simulink model "Sim4"  (R2014a)
settings: Solver=ode45  StartTime=0.0  StopTime=10.0  RelTol=1e-3
settings Model: Creator=OCAC  LastModifiedBy=OCAC

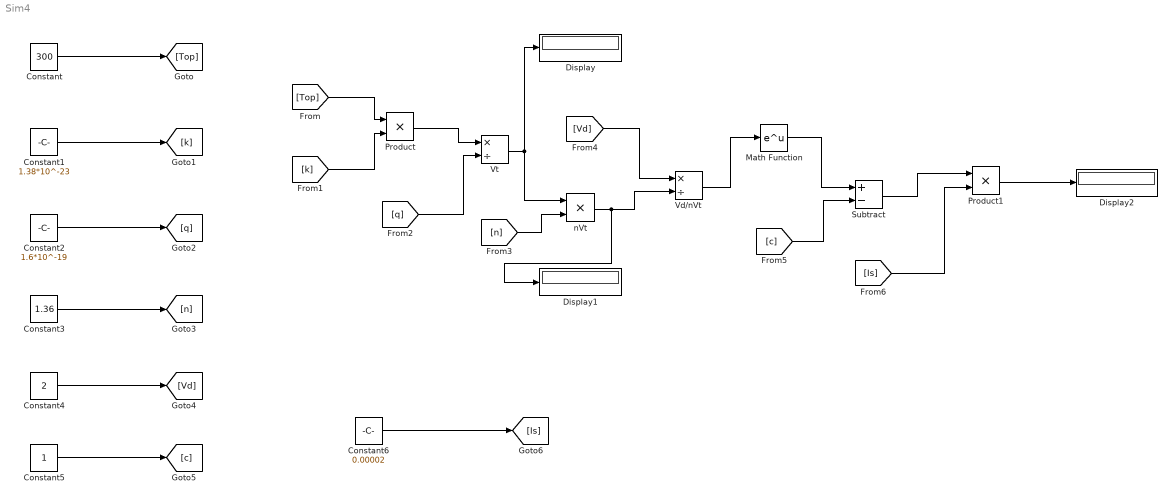
== system Sim4 ==
  Constant : Constant  Value=300
  Constant1 : Constant  Value=1.38*10^-23
  Constant2 : Constant  Value=1.6*10^-19
  Constant3 : Constant  Value=1.36
  Constant4 : Constant  Value=2
  Constant5 : Constant
  Constant6 : Constant  Value=0.00002
  Display : Display
  Display1 : Display
  Display2 : Display
  Math Function : Math  SaturateOnIntegerOverflow=on
  Product : Product
  Product1 : Product
  Subtract : Sum  Inputs=+-
  Vd/nVt : Product  Inputs=*/
  Vt : Product  Inputs=*/
  nVt : Product
  wires:
  Constant/1 -> [Top]
  Constant1/1 -> [k]
  Constant2/1 -> [q]
  [Top] -> Product/1
  [k] -> Product/2
  Product/1 -> Vt/1
  [q] -> Vt/2
  Vt/1 -> nVt/1, Display/1
  Constant3/1 -> [n]
  [n] -> nVt/2
  Constant4/1 -> [Vd]
  [Vd] -> Vd/nVt/1
  nVt/1 -> Display1/1, Vd/nVt/2
  Vd/nVt/1 -> Math Function/1
  Constant5/1 -> [c]
  Math Function/1 -> Subtract/1
  [c] -> Subtract/2
  Constant6/1 -> [Is]
  Subtract/1 -> Product1/1
  [Is] -> Product1/2
  Product1/1 -> Display2/1
